simulink model "uvms"  (Simulink 7.9)
settings: Solver=FixedStepDiscrete  StartTime=0.0  StopTime=10.0  RelTol=1e-3
values from neighbouring files (symbols this model uses):
  aq = [0,3,0,0,0,1]    [init.m]
  DH = struct('a',zeros(n,1),'d',zeros(n,1),'alpha',zeros(n,1))    [init.m]
  g0b = eye(4)    [init.m]
settings Model: Creator=simena  LastModifiedBy=simena
settings DebuggingCC: UnderspecifiedInitializationDetection=Simplified

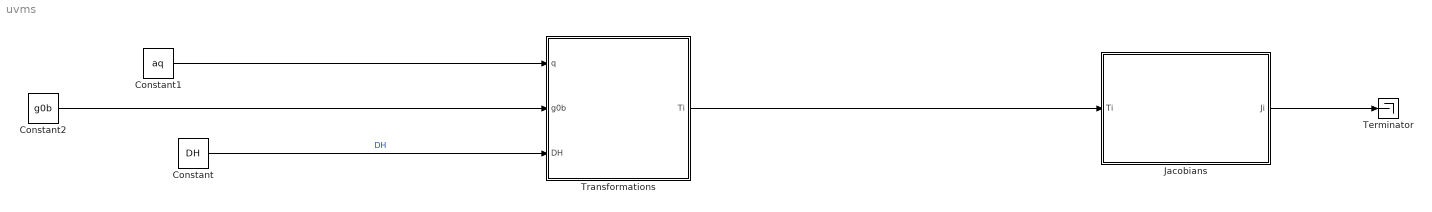
== system uvms ==
  Constant : Constant  Value=DH  OutDataTypeStr=Bus: slBus1
  Constant1 : Constant  Value=aq
  Constant2 : Constant  Value=g0b
  Jacobians : MATLAB Function  TreatAsAtomicUnit=on
  Terminator : Terminator
  Transformations : MATLAB Function  TreatAsAtomicUnit=on
  wires:
  Constant/1 -> Transformations/3(DH)  "DH"
  Constant1/1 -> Transformations/1(q)
  Transformations/1(Ti) -> Jacobians/1(Ti)
  Jacobians/1(Ji) -> Terminator/1
  Constant2/1 -> Transformations/2(g0b)

== matlab function Jacobians ==
  data: Ti input double; Ji output Bus: slBus3
function Ji = getJacobians(Ti)
%#codegen
    
    n=6;
    Ji = struct('Ji',zeros(n,n+6));
    ji=zeros(6,6)
    for i=1:n
        ji=getji(Ti,i);
        Ji.Ji(:,:,i) = [Ti.Adgbi_inv(:,:,i), Ti.Adgbi_inv(:,:,i)*ji];
    end
    
    j6=getje(Ti);
    Ji.Je=[Ti.Adgbe_inv, Ti.Adgbe_inv*j6];
    
end




% return matrix Ji (see report)
function mat = getji(Ti,i)
    n=6;
    mat=zeros(6,6);
    Xii=[0,0,0,0,0,1]';
    for j=1:n
        if j<=i
            mat(:,j) = Ti.Adg0i(:,:,i)*Xii;
        end
    end

end

% return matrix Ji (see report)
function mat = getje(Ti)
    n=6;
    mat=zeros(6,6);
    Xii=[0,0,0,0,0,1]';
    for i=1:(n-1)
        mat(:,i) = Ti.Adg0i(:,:,i)*Xii;
    end
    mat(:,6) = Ti.Adg0e*Xii;

end

== matlab function Transformations ==
  data: q input double; g0b input double; DH input double; Ti output Bus: slBus2
function Ti = getTransformations(q,g0b,DH)
%#codegen
% Return transformations, rotations, positions and adjoint matrices for
% robot links
% Tbi.gbi(:,:,i) is the transformation from b to i etc
    n=6;    % number of links
    Ti = struct('g0b',zeros(3,3),'g0i',zeros(4,4,n),'R0i', zeros(3,3,n),'p0i', zeros(3,1,n),  'Adg0i',zeros(6,6,n),'Adg0i_inv',zeros(6,6,n),   ...
    'gbi',zeros(4,4,n),'Rbi', zeros(3,3,n),'pbi', zeros(3,1,n),'Adgbi',zeros(6,6,n),'Adgbi_inv',zeros(6,6,n),...
    'g6e',eye(4) ,'g0e',zeros(4,4),'R0e', zeros(3,3),'p0e', zeros(3,1),  'Adg0e',zeros(6,6),'Adg0e_inv',zeros(6,6),   ...
    'gbe',zeros(4,4),'Rbe', zeros(3,3),'pbe', zeros(3,1),'Adgbe',zeros(6,6),'Adgbe_inv',zeros(6,6) ...
    );

    % initial matrices 
    g=eye(4);
    g0=g0b;
    
    % transformation from 0 and b to frame i
    for i=1:n
       Ti.gbi(:,:,i) = g*getHom(q,DH,i);
       Ti.Rbi(:,:,i) = getRot(Ti.gbi(:,:,i));
       Ti.pbi(:,:,i) = getPos(Ti.gbi(:,:,i));
       Ti.Adgbi(:,:,i) = getAdgbi(Ti.Rbi(:,:,i), Ti.pbi(:,:,i) );
       Ti.Adgbi_inv(:,:,i) = getAdgbi_inv(Ti.Rbi(:,:,i), Ti.pbi(:,:,i) );
       g=Ti.gbi(:,:,i);
       
       Ti.g0i(:,:,i) = g0*getHom(q,DH,i);
       Ti.R0i(:,:,i) = getRot(Ti.g0i(:,:,i));
       Ti.p0i(:,:,i) = getPos(Ti.g0i(:,:,i));
       Ti.Adg0i(:,:,i) = getAdgbi(Ti.R0i(:,:,i), Ti.p0i(:,:,i) );
       Ti.Adg0i_inv(:,:,i) = getAdgbi_inv(Ti.R0i(:,:,i), Ti.p0i(:,:,i) );
       g0=Ti.g0i(:,:,i);
    end
    
    % transformation from frame 0 to ee
    g0e = Ti.g0i(:,:,6)*Ti.g6e;
    Ti.g0e(:,:,i) = g0e;
    Ti.R0e(:,:,i) = getRot(g0e);
    Ti.p0e(:,:,i) = getPos(g0e);
    Ti.Adg0e(:,:,i) = getAdgbi(Ti.R0e(:,:,i), Ti.p0e(:,:,i) );
    Ti.Adg0e_inv(:,:,i) = getAdgbi_inv(Ti.R0e(:,:,i), Ti.p0e(:,:,i) );
    
    % transformation from frame b to ee
    gbe = Ti.gbi(:,:,6)*Ti.g6e;
    Ti.gbe(:,:,i) = gbe;
    Ti.Rbe(:,:,i) = getRot(gbe);
    Ti.pbe(:,:,i) = getPos(gbe);
    Ti.Adgbe(:,:,i) = getAdgbi(Ti.Rbe(:,:,i), Ti.pbe(:,:,i) );
    Ti.Adgbe_inv(:,:,i) = getAdgbi_inv(Ti.Rbe(:,:,i), Ti.pbe(:,:,i) );
    
    
    

end



% homogenous transformation matrix - DH convention
% mat=Rot_z(theta)Trans_z(d)Trans_x(a)Rot_x(alpha)
function mat=getHom(q,DH,i)
    alpha=DH.alpha(i);
    a=DH.a(i);
    d=DH.d(i);
    theta=q(i);
    mat=eye(4);
    mat=[cos(theta), -sin(theta)*cos(alpha), sin(theta)*sin(alpha), a*cos(theta);
         sin(theta), cos(theta)*cos(alpha), -cos(theta)*sin(alpha), a*sin(theta);
         0, sin(alpha), cos(alpha), d;
         0,0,0,1
    ];

end

% extract position from homogenous 
% matrix
function vec = getPos(g)
    vec=g(1:3,4);

end

% extract rotation matrix-part out of
% homogenous matrix
function mat = getRot(g)
    mat=g(1:3,1:3);
end


function mat = getAdgbi(R,p)
    mat = zeros(6,6);
    ps=skew(p);
    mat=[R , ps*R ; zeros(3,3), R ];
end

function mat = getAdgbi_inv(R,p)
    mat = zeros(6,6);
    Rt=transpose(R);
    ps=skew(p);
    mat=[Rt , -Rt*ps ; zeros(3,3), Rt ];
end

% return the skew symmetric matrix representation
% of vector
function mat = skew(vec)
    mat=[0, -vec(3), vec(2) ; vec(3), 0,vec(1); -vec(2), vec(1), 0];
end
